simulink model "sampleModel1632"  (R2023a)
settings: Solver=VariableStepAuto  StartTime=0.0  StopTime=10.0  RelTol=1e-3
libraries: hdlsllib x8
settings Model: Creator=user1  LastModifiedBy=user1

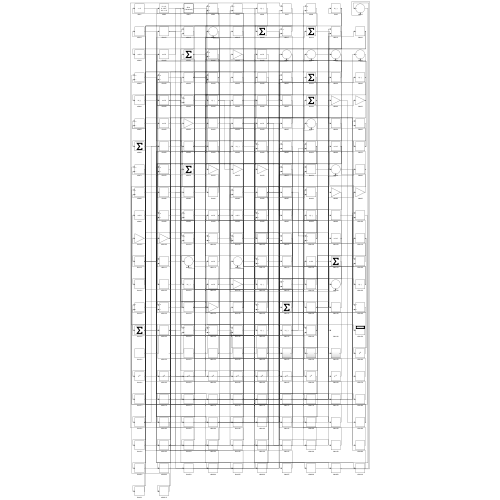
[thumbnail: Simulink's stored preview of the top-level diagram]
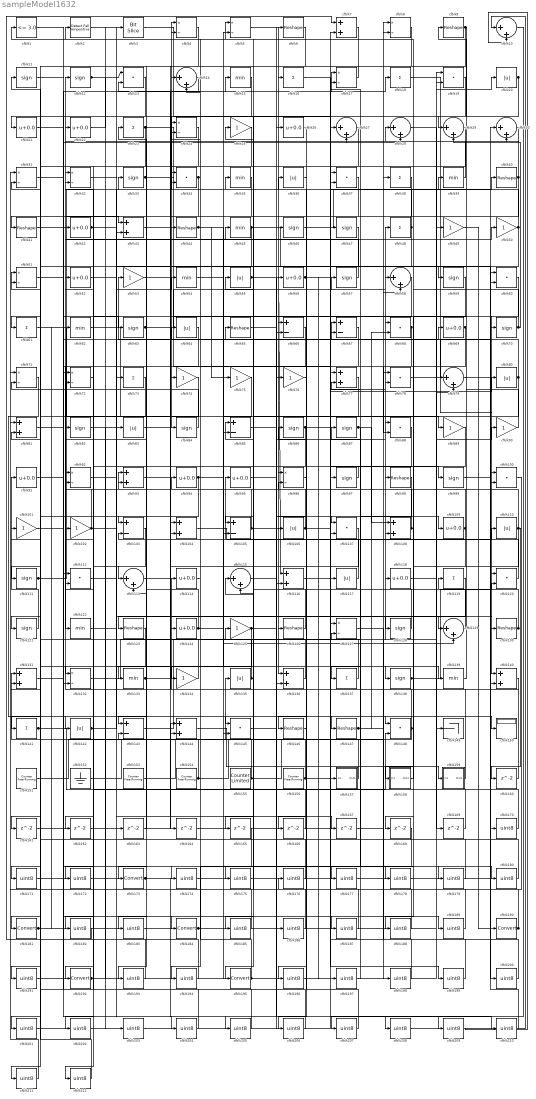
== system sampleModel1632 ==
  cfblk1 : hdlsllib/Logic and Bit Operations/Compare To Constant  relop=<=  const=3.0  OutDataTypeStr=boolean
  cfblk{10,14,27..30,58,79,113,115,129} (11 alike) : Sum  Inputs=|++
  cfblk{13,19,34,37,60,68,78,88,100,107,112,120,145,148} (14 alike) : DotProduct  OutDataTypeStr=Inherit: Inherit via internal rule
  cfblk{25,49..50,53,74..76,89..90,101..102,125,134} (13 alike) : Gain
  cfblk{66..67,85,103,105,143} (6 alike) : Sum  Inputs=+-
  cfblk{7,43,77,81,93,104,108,116,131,136,140,144} (12 alike) : Sum
  cfblk{20,36,55,64,80,83,106,110,117,135,142} (11 alike) : Abs  SaturateOnIntegerOverflow=off
  cfblk{21..22,26,42,52,56,69,91,94..95,109,114,118,124} (14 alike) : Bias  Bias=0.0  SaturateOnIntegerOverflow=off
  cfblk{11..12,33,46..47,57,59,63,70,82,84,86..87,97,99,111,121,128,138} (19 alike) : Signum
  cfblk{16,18,23,38,48,61,73,119,137,141} (10 alike) : Sum  Inputs=+
  cfblk{15,35,39,45,54,62,122,133,139} (9 alike) : MinMax
  cfblk{6,9,40..41,44,65,98,123,126,130,146..147} (12 alike) : Reshape
  cfblk{4..5,8,17,24,31..32,51,71..72,92,96,127,132} (14 alike) : Product  Inputs=*/  RndMeth=Zero  SaturateOnIntegerOverflow=on
  cfblk149 : Terminator
  cfblk150 : Display
  cfblk{151,153..154,156} (4 alike) : hdlsllib/Sources/Counter Free-Running  NumBits=16  tsamp=-1
  cfblk152 : Ground
  cfblk155 : hdlsllib/Sources/Counter Limited  uplimit=7  tsamp=-1
  cfblk157 : Subsystem
      settings: LibrarySourceBlock=|
      | hdlsllib/Ports &
      | Subsystems/Subsystem
  cfblk158 : Subsystem
      settings: LibrarySourceBlock=|
      | hdlsllib/Ports &
      | Subsystems/Subsystem
  cfblk159 : Subsystem
      settings: LibrarySourceBlock=|
      | hdlsllib/Ports &
      | Subsystems/Subsystem
  cfblk{160..169} (10 alike) : Delay  SampleTime=1
  cfblk{170..172,174..180,182..183,185..189,191,193..194,196..212} (37 alike) : DataTypeConversion  OutDataTypeStr=uint8  SaturateOnIntegerOverflow=off  RndMeth=Floor
  cfblk{173,181,184,190,192,195} (6 alike) : DataTypeConversion  SaturateOnIntegerOverflow=off  RndMeth=Floor
  cfblk2 : hdlsllib/Logic and Bit Operations/Detect Fall Nonpositive  vinit=0  OutDataTypeStr=boolean
  cfblk3 : hdlsllib/Logic and Bit Operations/Bit Slice  lidx=7  ridx=0
  wires:
  cfblk105/1 -> cfblk107/1, cfblk92/2
  cfblk102/1 -> cfblk33/1, cfblk34/1
  cfblk5/1 -> cfblk136/1
  cfblk64/1 -> cfblk123/1
  cfblk140/1 -> cfblk12/1
  cfblk159/1(Out1) -> cfblk114/1
  cfblk72/1 -> cfblk192/1
  cfblk61/1 -> cfblk89/1
  cfblk55/1 -> cfblk116/1, cfblk109/1
  cfblk18/1 -> cfblk140/1
  cfblk62/1 -> cfblk157/1(In1)
  cfblk15/1 -> cfblk84/1
  cfblk66/1 -> cfblk74/1
  cfblk28/1 -> cfblk149/1
  cfblk32/1 -> cfblk148/1
  cfblk156/1 -> cfblk69/1, cfblk131/2
  cfblk41/1 -> cfblk43/1
  cfblk90/1 -> cfblk22/1
  cfblk111/1 -> cfblk50/1, cfblk64/1, cfblk189/1
  cfblk25/1 -> cfblk143/1
  cfblk48/1 -> cfblk35/1, cfblk185/1
  cfblk106/1 -> cfblk24/2, cfblk199/1
  cfblk22/1 -> cfblk3/1
  cfblk19/1 -> cfblk66/1
  cfblk35/1 -> cfblk103/1
  cfblk69/1 -> cfblk122/1, cfblk132/2
  cfblk77/1 -> cfblk195/1
  cfblk130/1 -> cfblk87/1, cfblk1/1
  cfblk139/1 -> cfblk9/1
  cfblk121/1 -> cfblk91/1
  cfblk107/1 -> cfblk136/2
  cfblk141/1 -> cfblk148/2, cfblk28/2
  cfblk85/1 -> cfblk56/1
  cfblk67/1 -> cfblk92/1
  cfblk152/1 -> cfblk66/2
  cfblk96/1 -> cfblk36/1
  cfblk20/1 -> cfblk43/2, cfblk165/1
  cfblk83/1 -> cfblk17/1
  cfblk143/1 -> cfblk150/1
  cfblk49/1 -> cfblk190/1
  cfblk117/1 -> cfblk93/1
  cfblk137/1 -> cfblk125/1
  cfblk124/1 -> cfblk82/1, cfblk128/1
  cfblk60/1 -> cfblk120/1
  cfblk108/1 -> cfblk32/1, cfblk28/1
  cfblk138/1 -> cfblk120/2, cfblk90/1
  cfblk84/1 -> cfblk51/1
  cfblk12/1 -> cfblk13/1, cfblk163/1
  cfblk97/1 -> cfblk96/1
  cfblk17/1 -> cfblk16/1
  cfblk86/1 -> cfblk80/1, cfblk78/2, cfblk130/1, cfblk172/1
  cfblk2/1 -> cfblk129/1
  cfblk132/1 -> cfblk48/1
  cfblk126/1 -> cfblk85/1
  cfblk50/1 -> cfblk4/1, cfblk212/1
  cfblk144/1 -> cfblk159/1(In1)
  cfblk87/1 -> cfblk137/1, cfblk108/1
  cfblk70/1 -> cfblk2/1, cfblk30/2
  cfblk146/1 -> cfblk96/2
  cfblk7/1 -> cfblk181/1
  cfblk128/1 -> cfblk55/1
  cfblk113/1 -> cfblk15/1
  cfblk123/1 -> cfblk133/1
  cfblk80/1 -> cfblk53/1, cfblk146/1
  cfblk57/1 -> cfblk32/2
  cfblk147/1 -> cfblk38/1, cfblk68/2
  cfblk158/1(Out1) -> cfblk118/1
  cfblk9/1 -> cfblk29/1, cfblk183/1
  cfblk23/1 -> cfblk97/1, cfblk61/1
  cfblk120/1 -> cfblk95/1
  cfblk6/1 -> cfblk41/1
  cfblk157/1(Out1) -> cfblk135/1
  cfblk88/1 -> cfblk106/1
  cfblk71/1 -> cfblk142/1
  cfblk135/1 -> cfblk23/1, cfblk25/1
  cfblk148/1 -> cfblk67/1, cfblk143/2, cfblk98/1
  cfblk33/1 -> cfblk70/1, cfblk60/2
  cfblk63/1 -> cfblk58/1, cfblk116/2
  cfblk31/1 -> cfblk184/1
  cfblk116/1 -> cfblk40/1
  cfblk68/1 -> cfblk105/1, cfblk88/2
  cfblk104/1 -> cfblk110/1
  cfblk14/1 -> cfblk13/2
  cfblk52/1 -> cfblk59/1
  cfblk78/1 -> cfblk30/1
  cfblk122/1 -> cfblk54/1
  cfblk24/1 -> cfblk113/1
  cfblk151/1 -> cfblk8/2
  cfblk51/1 -> cfblk18/1
  cfblk8/1 -> cfblk21/1
  cfblk1/1 -> cfblk63/1
  cfblk75/1 -> cfblk105/2
  cfblk59/1 -> cfblk158/1(In1)
  cfblk110/1 -> cfblk4/2, cfblk160/1, cfblk178/1
  cfblk153/1 -> cfblk76/1
  cfblk36/1 -> cfblk126/1
  cfblk136/1 -> cfblk51/2
  cfblk94/1 -> cfblk57/1, cfblk211/1
  cfblk93/1 -> cfblk104/2
  cfblk134/1 -> cfblk103/2
  cfblk73/1 -> cfblk132/1
  cfblk37/1 -> cfblk173/1
  cfblk154/1 -> cfblk131/1, cfblk6/1
  cfblk53/1 -> cfblk45/1
  cfblk40/1 -> cfblk5/1, cfblk44/1
  cfblk11/1 -> cfblk145/1
  cfblk142/1 -> cfblk68/1, cfblk203/1
  cfblk45/1 -> cfblk140/2, cfblk171/1
  cfblk125/1 -> cfblk141/1, cfblk108/2
  cfblk129/1 -> cfblk119/1
  cfblk56/1 -> cfblk99/1, cfblk197/1
  cfblk39/1 -> cfblk24/1
  cfblk92/1 -> cfblk73/1
  cfblk42/1 -> cfblk138/1, cfblk134/1
  cfblk34/1 -> cfblk121/1, cfblk14/2
  cfblk74/1 -> cfblk111/1
  cfblk46/1 -> cfblk39/1
  cfblk3/1 -> cfblk47/1
  cfblk44/1 -> cfblk139/1, cfblk75/1
  cfblk155/1 -> cfblk94/1, cfblk67/2
  cfblk54/1 -> cfblk129/2
  cfblk109/1 -> cfblk17/2, cfblk168/1
  cfblk30/1 -> cfblk29/2
  cfblk114/1 -> cfblk14/1
  cfblk131/1 -> cfblk65/1
  cfblk95/1 -> cfblk88/1
  cfblk4/1 -> cfblk144/2
  cfblk133/1 -> cfblk20/1, cfblk147/1
  cfblk160/1 -> cfblk104/1
  cfblk13/1 -> cfblk161/1
  cfblk161/1 -> cfblk144/1
  cfblk29/1 -> cfblk162/1
  cfblk162/1 -> cfblk58/2
  cfblk163/1 -> cfblk113/2
  cfblk43/1 -> cfblk164/1
  cfblk164/1 -> cfblk85/2
  cfblk47/1 -> cfblk166/1
  cfblk166/1 -> cfblk93/2
  cfblk82/1 -> cfblk167/1
  cfblk167/1 -> cfblk8/1
  cfblk118/1 -> cfblk169/1
  cfblk169/1 -> cfblk52/1
  cfblk79/1 -> cfblk170/1
  cfblk170/1 -> cfblk124/1
  cfblk171/1 -> cfblk79/1
  cfblk172/1 -> cfblk79/2
  cfblk173/1 -> cfblk5/2, cfblk209/1
  cfblk21/1 -> cfblk174/1
  cfblk174/1 -> cfblk37/1
  cfblk168/1 -> cfblk175/1
  cfblk175/1 -> cfblk37/2
  cfblk100/1 -> cfblk176/1
  cfblk176/1 -> cfblk102/1
  cfblk98/1 -> cfblk177/1
  cfblk177/1 -> cfblk100/1
  cfblk178/1 -> cfblk100/2
  cfblk101/1 -> cfblk179/1
  cfblk179/1 -> cfblk19/1
  cfblk16/1 -> cfblk180/1
  cfblk180/1 -> cfblk101/1
  cfblk181/1 -> cfblk19/2, cfblk62/1
  cfblk58/1 -> cfblk182/1
  cfblk182/1 -> cfblk7/1
  cfblk183/1 -> cfblk7/2
  cfblk184/1 -> cfblk46/1, cfblk107/2
  cfblk185/1 -> cfblk31/1
  cfblk145/1 -> cfblk186/1
  cfblk186/1 -> cfblk31/2
  cfblk115/1 -> cfblk187/1
  cfblk187/1 -> cfblk71/2
  cfblk89/1 -> cfblk188/1
  cfblk188/1 -> cfblk115/1
  cfblk189/1 -> cfblk115/2
  cfblk190/1 -> cfblk42/1, cfblk71/1
  cfblk38/1 -> cfblk191/1
  cfblk191/1 -> cfblk49/1
  cfblk192/1 -> cfblk145/2, cfblk83/1
  cfblk119/1 -> cfblk193/1
  cfblk193/1 -> cfblk72/1
  cfblk165/1 -> cfblk194/1
  cfblk194/1 -> cfblk72/2
  cfblk195/1 -> cfblk34/2, cfblk117/1
  cfblk76/1 -> cfblk196/1
  cfblk196/1 -> cfblk77/1
  cfblk197/1 -> cfblk77/2
  cfblk127/1 -> cfblk198/1
  cfblk198/1 -> cfblk78/1
  cfblk199/1 -> cfblk127/1
  cfblk99/1 -> cfblk200/1
  cfblk200/1 -> cfblk127/2
  cfblk27/1 -> cfblk201/1
  cfblk201/1 -> cfblk26/1
  cfblk103/1 -> cfblk202/1
  cfblk202/1 -> cfblk27/1
  cfblk203/1 -> cfblk27/2
  cfblk112/1 -> cfblk204/1
  cfblk204/1 -> cfblk11/1
  cfblk91/1 -> cfblk205/1
  cfblk205/1 -> cfblk112/1
  cfblk26/1 -> cfblk206/1
  cfblk206/1 -> cfblk112/2
  cfblk10/1 -> cfblk207/1
  cfblk207/1 -> cfblk86/1
  cfblk65/1 -> cfblk208/1
  cfblk208/1 -> cfblk10/1
  cfblk209/1 -> cfblk10/2
  cfblk81/1 -> cfblk210/1
  cfblk210/1 -> cfblk60/1
  cfblk211/1 -> cfblk81/1
  cfblk212/1 -> cfblk81/2

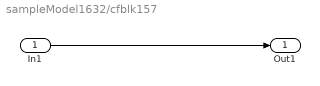
== system sampleModel1632/cfblk157 ==
  In1 : Inport
  Out1 : Outport
  wires:
  In1/1 -> Out1/1

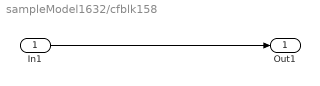
== system sampleModel1632/cfblk158 ==
  In1 : Inport
  Out1 : Outport
  wires:
  In1/1 -> Out1/1

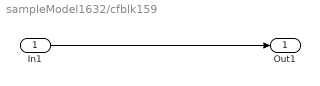
== system sampleModel1632/cfblk159 ==
  In1 : Inport
  Out1 : Outport
  wires:
  In1/1 -> Out1/1
